simulink model "bicycle"  (R2020a)
settings: Solver=VariableStepAuto  StartTime=0.0  StopTime=inf  FixedStep=0.1  RelTol=1e-3
model workspace (MAT data in the model file):
  Circuit = [89.6948814847 3.15970028499 1.18584712048 1.564238973 17.4007482574 16.7294379124 6.35282412808 8.85255180573 31.5089803119 1.04386532257 9.39692898789 18.2444675855 ... (2151 elements, 717x3)]
values from neighbouring files (symbols this model uses):
  A = 1    [PSO.m]    (also in init.m; matlab2.mat = 0.8)
  a = Circuit(:,1)    [PSO.m]    (also in init.m; matlab2.mat = [89.6948814847 3.15970028499 1.18584712048 1.564238973 17.40)
  b = Circuit(:,2)    [PSO.m]    (also in SpeedBar.m = bar(days,conc,0.4); init.m; matlab2.mat = [0 0.0943959490766 -0.00625094781681 0.00830452466906 0.0231)
  c = Circuit(:,3)    [PSO.m]    (also in init.m; matlab2.mat = [0 0.0367353 0.0664904 0.2161644 0.4182007 0.4447518 0.46434)
  Cd = 0.2    [PSO.m]    (also in init.m; matlab2.mat = 0.235)
  efficiency = 0.98    [PSO.m]    (also in init.m; matlab2.mat)
  k1 = x(j,1)    [PSO.m]    (also in PSO_road.m = k1_PSO; init.m = 0.0112626977304; matlab2.mat = 0.00872664625997)
  k2 = x(j,2)    [PSO.m]    (also in PSO_road.m = k2_PSO; init.m = -0.495769209118; matlab2.mat = -0.5)
  k3 = x(j,3)    [PSO.m]    (also in PSO_road.m = k3_PSO; init.m = 0.0700919071468; matlab2.mat = 0.07)
  k4 = x(j,4)    [PSO.m]    (also in PSO_road.m = k4_PSO; init.m = -1.40513990779; matlab2.mat = -1.39)
  m = 9.5+55    (= 64.5)    [PSO.m]    (also in init.m; matlab2.mat)
  mu = 0.012    [PSO.m]    (also in init.m; matlab2.mat)
  phi = 0.85    [PSO.m]    (also in init.m; matlab2.mat)
  r = 0.6096/2    (= 0.3048)    [PSO.m]    (also in init.m; matlab2.mat; road.m = num(i,1))
  ro = 1.2258    [PSO.m]    (also in init.m; matlab2.mat = 1.1258)
  v0 = 1    [PSO.m]    (also in init.m; matlab2.mat)
  wind_direction = 0    [PSO.m]    (also in init.m)
  wind_speed = 0    [PSO.m]    (also in init.m)
settings Model: OrderedModelArguments=off  Creator=Technic  LastModifiedBy=ZRG
settings SolverCC: MaxConsecutiveZCs=100000  ZeroCrossAlgorithm=Adaptive
settings DebuggingCC: IgnoredZcDiagnostic=none

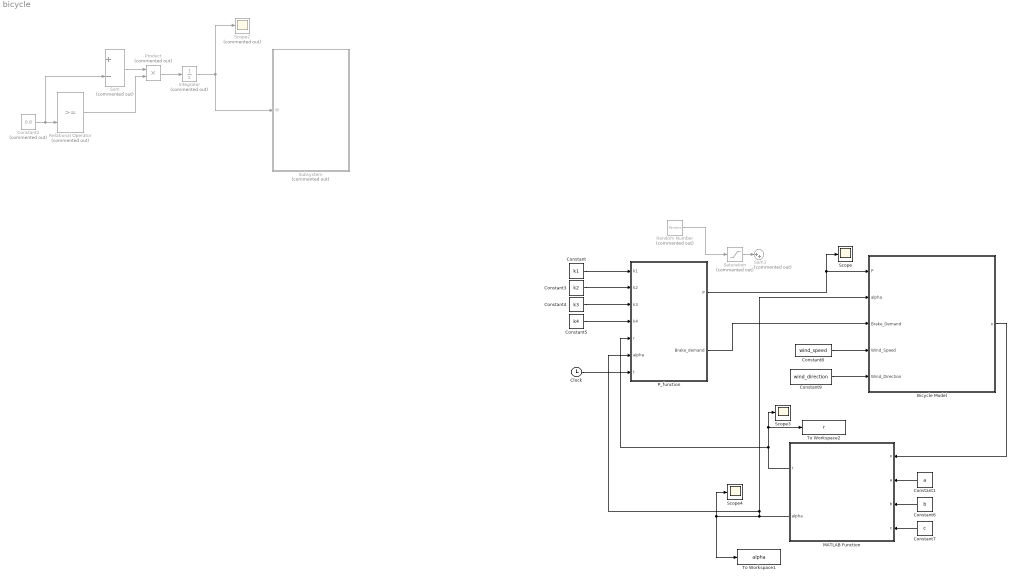
== system bicycle ==
  Bicycle Model : Subsystem
  Clock : Clock
  Constant : Constant  Value=k1
  Constant1 : Constant  Value=a
  Constant2 : Constant  Commented=on  Value=0.8
  Constant3 : Constant  Value=k2
  Constant4 : Constant  Value=k3
  Constant5 : Constant  Value=k4
  Constant6 : Constant  Value=b
  Constant7 : Constant  Value=c
  Constant8 : Constant  Value=wind_speed
  Constant9 : Constant  Value=wind_direction
  Integrator : Integrator  Commented=on
  MATLAB Function : MATLAB Function  TreatAsAtomicUnit=on
  P_function : MATLAB Function  TreatAsAtomicUnit=on
  Product : Product  Commented=on
  Random Number : RandomNumber  Commented=on  Variance=0.2  SampleTime=50
  Relational Operator : RelationalOperator  Commented=on  OutDataTypeStr=boolean  RndMeth=Simplest
  Saturation : Saturate  Commented=on  UpperLimit=0.05  LowerLimit=-0.05
  Scope : Scope
  Scope2 : Scope  Commented=on
  Scope3 : Scope
  Scope4 : Scope
  Subsystem : Subsystem  Commented=on
  Sum : Sum  Commented=on  Inputs=+-
  Sum1 : Sum  Commented=on  Inputs=|++
  To Workspace1 : ToWorkspace  VariableName=alpha  SaveFormat=Timeseries  SampleTime=-1
  To Workspace2 : ToWorkspace  VariableName=r  SaveFormat=Timeseries  SampleTime=-1
  wires:
  P_function/2(Brake_demand) -> Bicycle Model/3(Brake_Demand)
  Integrator/1 -> Scope2/1, Subsystem/1(W)
  Constant2/1 -> Sum/2, Relational Operator/2
  Sum/1 -> Product/1
  Relational Operator/1 -> Product/2
  Product/1 -> Integrator/1
  Clock/1 -> P_function/7(t)
  Constant/1 -> P_function/1(k1)
  Constant3/1 -> P_function/2(k2)
  Constant4/1 -> P_function/3(k3)
  Constant5/1 -> P_function/4(k4)
  Bicycle Model/1(x) -> MATLAB Function/1(x)
  MATLAB Function/1(r) -> To Workspace2/1, Scope3/1, P_function/5(r)
  MATLAB Function/2(alpha) -> P_function/6(alpha), Bicycle Model/2(alpha), To Workspace1/1, Scope4/1
  Constant1/1 -> MATLAB Function/2(a)
  Constant6/1 -> MATLAB Function/3(b)
  Constant7/1 -> MATLAB Function/4(c)
  Random Number/1 -> Saturation/1
  Saturation/1 -> Sum1/1
  P_function/1(P) -> Scope/1, Bicycle Model/1(P)
  Constant8/1 -> Bicycle Model/4(Wind_Speed)
  Constant9/1 -> Bicycle Model/5(Wind_Direction)

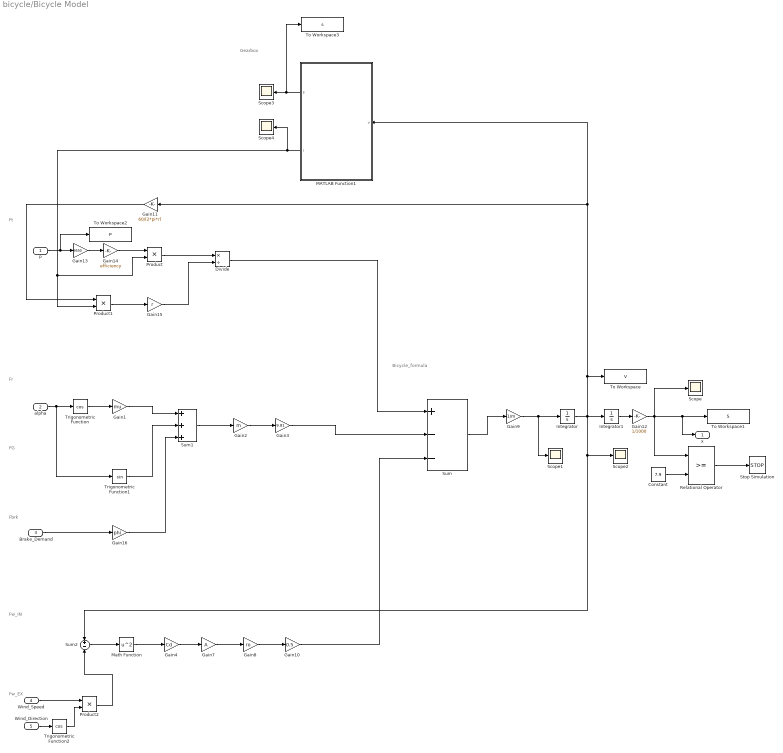
== system bicycle/Bicycle Model ==
  note: Gearbox
  note: Bicycle_formula
  note: Ft
  note: Fr
  note: FG
  note: Fw_IN
  note: Fbrk
  note: Fw_EX
  P : Inport
  alpha : Inport  Port=2
  Brake_Demand : Inport  Port=3
  Wind_Speed : Inport  Port=4
  Wind_Direction : Inport  Port=5
  Constant : Constant  Value=7.9
  Divide : Product  Inputs=*/
  Gain1 : Gain  Gain=mu
  Gain10 : Gain  Gain=0.5
  Gain11 : Gain  Gain=60/(2*pi*r)
  Gain12 : Gain  Gain=1/1000
  Gain13 : Gain  Gain=9550
  Gain14 : Gain  Gain=efficiency
  Gain15 : Gain  Gain=r
  Gain16 : Gain  Gain=phi
  Gain2 : Gain  Gain=m
  Gain3 : Gain  Gain=9.81
  Gain4 : Gain  Gain=Cd
  Gain7 : Gain  Gain=A
  Gain8 : Gain  Gain=ro
  Gain9 : Gain  Gain=1/m
  Integrator : Integrator  InitialCondition=v0
  Integrator1 : Integrator
  MATLAB Function1 : MATLAB Function  TreatAsAtomicUnit=on
  Math Function : Math  Operator=square  SaturateOnIntegerOverflow=on
  Product : Product
  Product1 : Product
  Product2 : Product
  Relational Operator : RelationalOperator  OutDataTypeStr=boolean  RndMeth=Simplest
  Scope{,1..4} (5 alike) : Scope
  Stop Simulation : Stop
  Sum : Sum  Inputs=+--
  Sum1 : Sum  Inputs=+++
  Sum2 : Sum  Inputs=+-
  To Workspace : ToWorkspace  VariableName=V  SaveFormat=Timeseries  SampleTime=-1
  To Workspace1 : ToWorkspace  VariableName=S  SaveFormat=Timeseries  SampleTime=-1
  To Workspace2 : ToWorkspace  VariableName=P  SaveFormat=Timeseries  SampleTime=-1
  To Workspace3 : ToWorkspace  VariableName=s  SaveFormat=Timeseries  SampleTime=-1
  Trigonometric Function : Trigonometry  Operator=cos
  Trigonometric Function1 : Trigonometry
  Trigonometric Function2 : Trigonometry  Operator=cos
  x : Outport
  wires:
  P/1 -> To Workspace2/1, Gain13/1
  alpha/1 -> Trigonometric Function1/1, Trigonometric Function/1
  Trigonometric Function/1 -> Gain1/1
  Gain2/1 -> Gain3/1
  Math Function/1 -> Gain4/1
  Gain4/1 -> Gain7/1
  Gain7/1 -> Gain8/1
  Gain3/1 -> Sum/2
  Sum/1 -> Gain9/1
  Gain9/1 -> Scope1/1, Integrator/1
  Integrator1/1 -> Gain12/1
  Gain8/1 -> Gain10/1
  Gain10/1 -> Sum/3
  Gain11/1 -> Product1/1
  Gain12/1 -> Relational Operator/1, x/1, To Workspace1/1, Scope/1
  Gain13/1 -> Gain14/1
  Gain14/1 -> Product/1
  MATLAB Function1/2(i) -> Product/2, Product1/2, Scope4/1
  Product/1 -> Divide/1
  Gain15/1 -> Divide/2
  Divide/1 -> Sum/1
  Product1/1 -> Gain15/1
  MATLAB Function1/1(s) -> To Workspace3/1, Scope3/1
  Integrator/1 -> MATLAB Function1/1(v), Gain11/1, To Workspace/1, Sum2/1, Scope2/1, Integrator1/1
  Relational Operator/1 -> Stop Simulation/1
  Constant/1 -> Relational Operator/2
  Brake_Demand/1 -> Gain16/1
  Sum1/1 -> Gain2/1
  Gain1/1 -> Sum1/1
  Trigonometric Function1/1 -> Sum1/2
  Gain16/1 -> Sum1/3
  Wind_Direction/1 -> Trigonometric Function2/1
  Wind_Speed/1 -> Product2/1
  Trigonometric Function2/1 -> Product2/2
  Sum2/1 -> Math Function/1
  Product2/1 -> Sum2/2

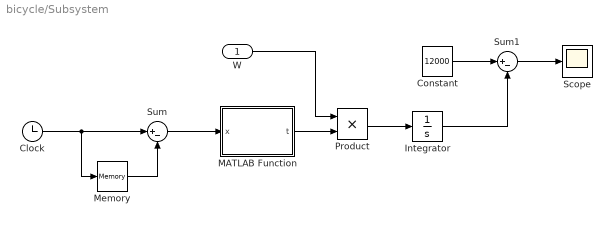
== system bicycle/Subsystem ==
  W : Inport
  Clock : Clock
  Constant : Constant  Value=12000
  Integrator : Integrator
  MATLAB Function : MATLAB Function  TreatAsAtomicUnit=on
  Memory : Memory
  Product : Product
  Scope : Scope
  Sum : Sum  Inputs=|+-
  Sum1 : Sum  Inputs=|+-
  wires:
  Clock/1 -> Memory/1, Sum/1
  Memory/1 -> Sum/2
  Sum/1 -> MATLAB Function/1(x)
  MATLAB Function/1(t) -> Product/2
  W/1 -> Product/1
  Product/1 -> Integrator/1
  Constant/1 -> Sum1/1
  Integrator/1 -> Sum1/2
  Sum1/1 -> Scope/1

== matlab function bicycle/P_function ==
  data: k1 input; P output; k2 input; k3 input; k4 input; r input; alpha input; t input; Brake_demand output
function [P, Brake_demand] = fcn(k1,k2,k3,k4,r,alpha,t)
    if t>10
        if alpha < -0.034 || r > 40
            Brake_demand=0.01;
            P=0;
        else
            Brake_demand=0;
            temp=k1*r + k2*alpha +k3*log(t)+k4;
            P = 1/(1+exp(-temp));
        end
    else
        Brake_demand=0;
        temp=k1*r + k2*alpha +k3*log(t)+k4;
        P = 1/(1+exp(-temp));
    end
end

== matlab function bicycle/Subsystem/MATLAB Function ==
  data: x input; t output
function t = fcn(x)
    t=exp(-x/377);
end

== matlab function bicycle/Bicycle Model/MATLAB Function1 ==
  data: v input; s output; i output
function [s, i]= fcn(v)
    s=0;
    i_total=[1.47 1.27 1.15 1 0.86 0.78 0.68];
    if v<5.77
        s=1;
    elseif v>=5.77 && v<6.67
        s=2;
    elseif v>=6.67 && v<7.37
        s=3;
    elseif v>=7.37 && v<8.48
        s=4;
    elseif v>=8.48 && v<9.86
        s=5;
    elseif v>=9.86 && v<10.87
        s=6;
    elseif v>=10.87
        s=7;
    end
    i=i_total(s);
end

== matlab function bicycle/MATLAB Function ==
  data: x input; r output; alpha output; a input; b input; c input
function [r,alpha] = road(x,a,b,c)
    n=length(c);
    if x<c(1)
        alpha=b(1);
        r=a(1);
    else
        for i = 1:n-1
            if x<c(i+1)
               alpha=b(i);
               r=a(i); 
               break;
            else
                alpha=b(n);
                r=a(n);
            end
        end
    end
end
